simulink model "test_Walk_In"  (R2014a)
settings: Solver=ode45  StartTime=0.0  StopTime=24*3600  RelTol=1e-3
libraries: refrigeration x1
settings Model: Creator=avenger  LastModifiedBy=avenger
settings OptimizationCC: SimCompilerOptimization=off
settings DebuggingCC: MergeDetectMultiDrivingBlocksExec=error  FrameProcessingCompatibilityMsg=error
settings RTWCC: RTWCompilerOptimization=off

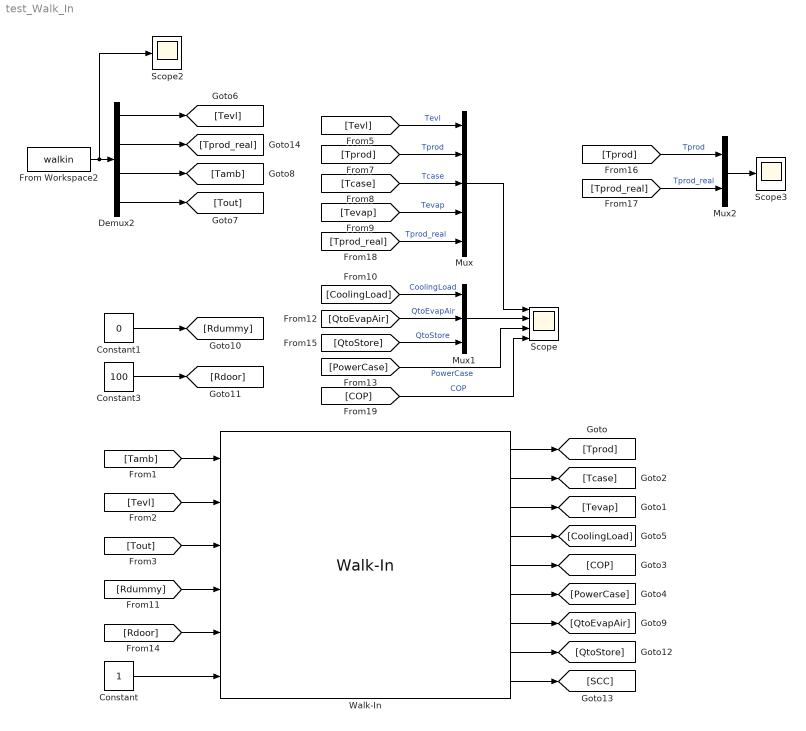
== system test_Walk_In ==
  Constant : Constant
  Constant1 : Constant  Value=0
  Constant3 : Constant  Value=100
  Demux2 : Demux
  From Workspace2 : FromWorkspace  VariableName=walkin  SampleTime=0
  Mux : Mux  Inputs=5
  Mux1 : Mux  Inputs=3
  Mux2 : Mux  Inputs=2
  Scope : Scope  NumInputPorts=4
      settings: ShowLegends=on  TimeRange=700000  YMin=-30~-10000~0~-5  YMax=40~10000~60~5
  Scope2 : Scope
      settings: ShowLegends=on  TimeRange=700000  YMin=-25  SaveName=ScopeData2
  Scope3 : Scope
      settings: ShowLegends=on  TimeRange=700000  YMin=-45  YMax=-10  SaveName=ScopeData3
  Walk-In : refrigeration/Refrigeration/Walk-In  Tcase_0=0  Tprod_0=0  Tevap_0=0  Cprod=9.6353e4  Rcase=9.6362e-2  Ccase=9.9033e5  Alpha=3.3139e-2  RatedLoad=4255  Qfan=329  Qlights=62  LHR=0  Cevap=400000  p_value=400
  wires:
  Walk-In/1 -> [Tprod]
  Walk-In/2 -> [Tcase]
  Walk-In/3 -> [Tevap]
  Walk-In/4 -> [CoolingLoad]
  [Tevl] -> Walk-In/2
  [Tout] -> Walk-In/3
  [Tamb] -> Walk-In/1
  Mux/1 -> Scope/1
  [Tevl] -> Mux/1  "Tevl"
  [Tcase] -> Mux/3  "Tcase"
  [Tevap] -> Mux/4  "Tevap"
  [Tprod] -> Mux/2  "Tprod"
  Mux1/1 -> Scope/2
  [QtoEvapAir] -> Mux1/2  "QtoEvapAir"
  [CoolingLoad] -> Mux1/1  "CoolingLoad"
  [PowerCase] -> Scope/3  "PowerCase"
  Constant/1 -> Walk-In/6
  [Rdoor] -> Walk-In/5
  [Rdummy] -> Walk-In/4
  Constant1/1 -> [Rdummy]
  Constant3/1 -> [Rdoor]
  [QtoStore] -> Mux1/3  "QtoStore"
  Walk-In/5 -> [COP]
  Walk-In/6 -> [PowerCase]
  Walk-In/7 -> [QtoEvapAir]
  Walk-In/8 -> [QtoStore]
  Walk-In/9 -> [SCC]
  Demux2/1 -> [Tevl]
  Demux2/2 -> [Tprod_real]
  Demux2/3 -> [Tamb]
  Demux2/4 -> [Tout]
  [Tprod_real] -> Mux2/2  "Tprod_real"
  [Tprod] -> Mux2/1  "Tprod"
  Mux2/1 -> Scope3/1
  [Tprod_real] -> Mux/5  "Tprod_real"
  [COP] -> Scope/4  "COP"
  From Workspace2/1 -> Scope2/1, Demux2/1
